simulink model "Rotor_Delevitation_PB_NonWhirl"  (R2024b)
settings: Solver=ode15s  StartTime=0.0  StopTime=.7  FixedStep=1e-4  MaxStep=1e-3  RelTol=1e-3  AbsTol=1e-3
undefined symbols (not defined in the file): points, X, x1, x2, x_i, x_o, Y, y_i, y_o, Z, z_i, z_o
libraries: sm_lib x361, nesl_utility x6
(part 4 of 6)

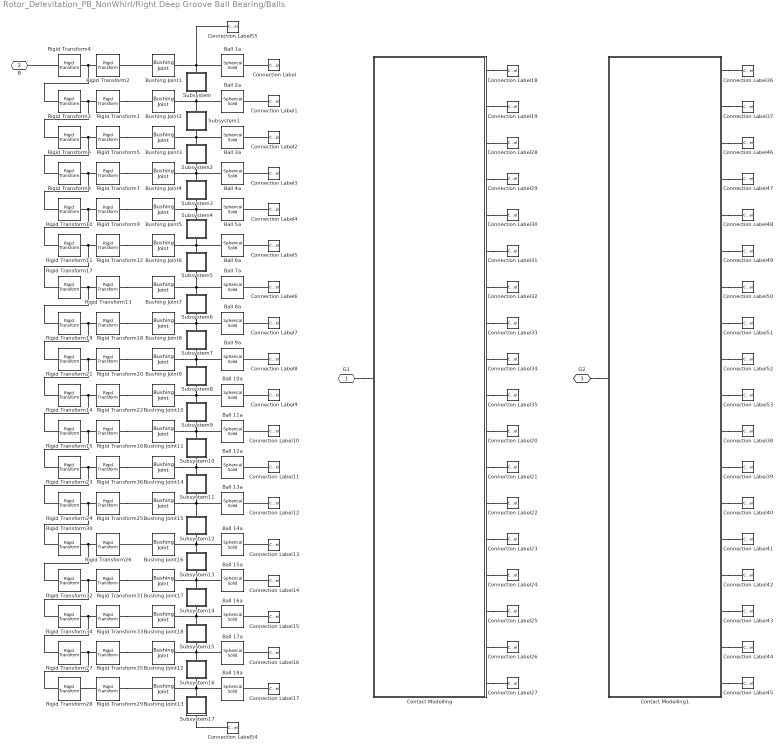
== system Rotor_Delevitation_PB_NonWhirl/Right Deep Groove Ball Bearing/Balls ==
  Ball 10a : sm_lib/Body Elements/Spherical Solid  SphereRadius=R-(C/2)  SphereRadiusUnits=mm  ExportEntireGeometry=on  InertiaType=CalculateFromGeometry  BasedOnType=Density  Density=1000  DensityUnits=kg/m^3  Mass=1  MassUnits=kg  CenterOfMass=[0 0 0]  CenterOfMassUnits=m  MomentsOfInertia=[1 1 1]  MomentsOfInertiaUnits=kg*m^2  ProductsOfInertia=[0 0 0]  ProductsOfInertiaUnits=kg*m^2  GraphicType=FromGeometry  MarkerShape=Sphere  MarkerSize=10  GraphicVisPropType=SimpleVisualProperties  GraphicDiffuseColor=[0.3922 0.8314 0.07451]  GraphicOpacity=1  GraphicSpecularColor=[0.5 0.5 0.5 1.0]  GraphicAmbientColor=[0.15 0.15 0.15 1.0]  GraphicEmissiveColor=[0.0 0.0 0.0 1.0]  GraphicShininess=75  DoExposeReferenceFrame=on  SerializedFrames=<Frames/>
  Ball 11a : sm_lib/Body Elements/Spherical Solid  SphereRadius=R-(C/2)  SphereRadiusUnits=mm  ExportEntireGeometry=on  InertiaType=CalculateFromGeometry  BasedOnType=Density  Density=1000  DensityUnits=kg/m^3  Mass=1  MassUnits=kg  CenterOfMass=[0 0 0]  CenterOfMassUnits=m  MomentsOfInertia=[1 1 1]  MomentsOfInertiaUnits=kg*m^2  ProductsOfInertia=[0 0 0]  ProductsOfInertiaUnits=kg*m^2  GraphicType=FromGeometry  MarkerShape=Sphere  MarkerSize=10  GraphicVisPropType=SimpleVisualProperties  GraphicDiffuseColor=[0.3922 0.8314 0.07451]  GraphicOpacity=1  GraphicSpecularColor=[0.5 0.5 0.5 1.0]  GraphicAmbientColor=[0.15 0.15 0.15 1.0]  GraphicEmissiveColor=[0.0 0.0 0.0 1.0]  GraphicShininess=75  DoExposeReferenceFrame=on  SerializedFrames=<Frames/>
  Ball 12a : sm_lib/Body Elements/Spherical Solid  SphereRadius=R-(C/2)  SphereRadiusUnits=mm  ExportEntireGeometry=on  InertiaType=CalculateFromGeometry  BasedOnType=Density  Density=1000  DensityUnits=kg/m^3  Mass=1  MassUnits=kg  CenterOfMass=[0 0 0]  CenterOfMassUnits=m  MomentsOfInertia=[1 1 1]  MomentsOfInertiaUnits=kg*m^2  ProductsOfInertia=[0 0 0]  ProductsOfInertiaUnits=kg*m^2  GraphicType=FromGeometry  MarkerShape=Sphere  MarkerSize=10  GraphicVisPropType=SimpleVisualProperties  GraphicDiffuseColor=[0.3922 0.8314 0.07451]  GraphicOpacity=1  GraphicSpecularColor=[0.5 0.5 0.5 1.0]  GraphicAmbientColor=[0.15 0.15 0.15 1.0]  GraphicEmissiveColor=[0.0 0.0 0.0 1.0]  GraphicShininess=75  DoExposeReferenceFrame=on  SerializedFrames=<Frames/>
  Ball 13a : sm_lib/Body Elements/Spherical Solid  SphereRadius=R-(C/2)  SphereRadiusUnits=mm  ExportEntireGeometry=on  InertiaType=CalculateFromGeometry  BasedOnType=Density  Density=1000  DensityUnits=kg/m^3  Mass=1  MassUnits=kg  CenterOfMass=[0 0 0]  CenterOfMassUnits=m  MomentsOfInertia=[1 1 1]  MomentsOfInertiaUnits=kg*m^2  ProductsOfInertia=[0 0 0]  ProductsOfInertiaUnits=kg*m^2  GraphicType=FromGeometry  MarkerShape=Sphere  MarkerSize=10  GraphicVisPropType=SimpleVisualProperties  GraphicDiffuseColor=[0.3922 0.8314 0.07451]  GraphicOpacity=1  GraphicSpecularColor=[0.5 0.5 0.5 1.0]  GraphicAmbientColor=[0.15 0.15 0.15 1.0]  GraphicEmissiveColor=[0.0 0.0 0.0 1.0]  GraphicShininess=75  DoExposeReferenceFrame=on  SerializedFrames=<Frames/>
  "Ball 14a " : sm_lib/Body Elements/Spherical Solid  SphereRadius=R-(C/2)  SphereRadiusUnits=mm  ExportEntireGeometry=on  InertiaType=CalculateFromGeometry  BasedOnType=Density  Density=1000  DensityUnits=kg/m^3  Mass=1  MassUnits=kg  CenterOfMass=[0 0 0]  CenterOfMassUnits=m  MomentsOfInertia=[1 1 1]  MomentsOfInertiaUnits=kg*m^2  ProductsOfInertia=[0 0 0]  ProductsOfInertiaUnits=kg*m^2  GraphicType=FromGeometry  MarkerShape=Sphere  MarkerSize=10  GraphicVisPropType=SimpleVisualProperties  GraphicDiffuseColor=[0.3922 0.8314 0.07451]  GraphicOpacity=1  GraphicSpecularColor=[0.5 0.5 0.5 1.0]  GraphicAmbientColor=[0.15 0.15 0.15 1.0]  GraphicEmissiveColor=[0.0 0.0 0.0 1.0]  GraphicShininess=75  DoExposeReferenceFrame=on  SerializedFrames=<Frames/>
  Ball 15a : sm_lib/Body Elements/Spherical Solid  SphereRadius=R-(C/2)  SphereRadiusUnits=mm  ExportEntireGeometry=on  InertiaType=CalculateFromGeometry  BasedOnType=Density  Density=1000  DensityUnits=kg/m^3  Mass=1  MassUnits=kg  CenterOfMass=[0 0 0]  CenterOfMassUnits=m  MomentsOfInertia=[1 1 1]  MomentsOfInertiaUnits=kg*m^2  ProductsOfInertia=[0 0 0]  ProductsOfInertiaUnits=kg*m^2  GraphicType=FromGeometry  MarkerShape=Sphere  MarkerSize=10  GraphicVisPropType=SimpleVisualProperties  GraphicDiffuseColor=[0.3922 0.8314 0.07451]  GraphicOpacity=1  GraphicSpecularColor=[0.5 0.5 0.5 1.0]  GraphicAmbientColor=[0.15 0.15 0.15 1.0]  GraphicEmissiveColor=[0.0 0.0 0.0 1.0]  GraphicShininess=75  DoExposeReferenceFrame=on  SerializedFrames=<Frames/>
  Ball 16a : sm_lib/Body Elements/Spherical Solid  SphereRadius=R-(C/2)  SphereRadiusUnits=mm  ExportEntireGeometry=on  InertiaType=CalculateFromGeometry  BasedOnType=Density  Density=1000  DensityUnits=kg/m^3  Mass=1  MassUnits=kg  CenterOfMass=[0 0 0]  CenterOfMassUnits=m  MomentsOfInertia=[1 1 1]  MomentsOfInertiaUnits=kg*m^2  ProductsOfInertia=[0 0 0]  ProductsOfInertiaUnits=kg*m^2  GraphicType=FromGeometry  MarkerShape=Sphere  MarkerSize=10  GraphicVisPropType=SimpleVisualProperties  GraphicDiffuseColor=[0.3922 0.8314 0.07451]  GraphicOpacity=1  GraphicSpecularColor=[0.5 0.5 0.5 1.0]  GraphicAmbientColor=[0.15 0.15 0.15 1.0]  GraphicEmissiveColor=[0.0 0.0 0.0 1.0]  GraphicShininess=75  DoExposeReferenceFrame=on  SerializedFrames=<Frames/>
  Ball 17a : sm_lib/Body Elements/Spherical Solid  SphereRadius=R-(C/2)  SphereRadiusUnits=mm  ExportEntireGeometry=on  InertiaType=CalculateFromGeometry  BasedOnType=Density  Density=1000  DensityUnits=kg/m^3  Mass=1  MassUnits=kg  CenterOfMass=[0 0 0]  CenterOfMassUnits=m  MomentsOfInertia=[1 1 1]  MomentsOfInertiaUnits=kg*m^2  ProductsOfInertia=[0 0 0]  ProductsOfInertiaUnits=kg*m^2  GraphicType=FromGeometry  MarkerShape=Sphere  MarkerSize=10  GraphicVisPropType=SimpleVisualProperties  GraphicDiffuseColor=[0.3922 0.8314 0.07451]  GraphicOpacity=1  GraphicSpecularColor=[0.5 0.5 0.5 1.0]  GraphicAmbientColor=[0.15 0.15 0.15 1.0]  GraphicEmissiveColor=[0.0 0.0 0.0 1.0]  GraphicShininess=75  DoExposeReferenceFrame=on  SerializedFrames=<Frames/>
  Ball 18a : sm_lib/Body Elements/Spherical Solid  SphereRadius=R-(C/2)  SphereRadiusUnits=mm  ExportEntireGeometry=on  InertiaType=CalculateFromGeometry  BasedOnType=Density  Density=1000  DensityUnits=kg/m^3  Mass=1  MassUnits=kg  CenterOfMass=[0 0 0]  CenterOfMassUnits=m  MomentsOfInertia=[1 1 1]  MomentsOfInertiaUnits=kg*m^2  ProductsOfInertia=[0 0 0]  ProductsOfInertiaUnits=kg*m^2  GraphicType=FromGeometry  MarkerShape=Sphere  MarkerSize=10  GraphicVisPropType=SimpleVisualProperties  GraphicDiffuseColor=[0.3922 0.8314 0.07451]  GraphicOpacity=1  GraphicSpecularColor=[0.5 0.5 0.5 1.0]  GraphicAmbientColor=[0.15 0.15 0.15 1.0]  GraphicEmissiveColor=[0.0 0.0 0.0 1.0]  GraphicShininess=75  DoExposeReferenceFrame=on  SerializedFrames=<Frames/>
  Ball 1a : sm_lib/Body Elements/Spherical Solid  SphereRadius=R-(C/2)  SphereRadiusUnits=mm  ExportEntireGeometry=on  InertiaType=CalculateFromGeometry  BasedOnType=Density  Density=1000  DensityUnits=kg/m^3  Mass=1  MassUnits=kg  CenterOfMass=[0 0 0]  CenterOfMassUnits=m  MomentsOfInertia=[1 1 1]  MomentsOfInertiaUnits=kg*m^2  ProductsOfInertia=[0 0 0]  ProductsOfInertiaUnits=kg*m^2  GraphicType=FromGeometry  MarkerShape=Sphere  MarkerSize=10  GraphicVisPropType=SimpleVisualProperties  GraphicDiffuseColor=[0.851 0.3255 0.09804]  GraphicOpacity=1  GraphicSpecularColor=[0.5 0.5 0.5 1.0]  GraphicAmbientColor=[0.15 0.15 0.15 1.0]  GraphicEmissiveColor=[0.0 0.0 0.0 1.0]  GraphicShininess=75  DoExposeReferenceFrame=on  SerializedFrames=<Frames/>
  Ball 2a : sm_lib/Body Elements/Spherical Solid  SphereRadius=R-(C/2)  SphereRadiusUnits=mm  ExportEntireGeometry=on  InertiaType=CalculateFromGeometry  BasedOnType=Density  Density=1000  DensityUnits=kg/m^3  Mass=1  MassUnits=kg  CenterOfMass=[0 0 0]  CenterOfMassUnits=m  MomentsOfInertia=[1 1 1]  MomentsOfInertiaUnits=kg*m^2  ProductsOfInertia=[0 0 0]  ProductsOfInertiaUnits=kg*m^2  GraphicType=FromGeometry  MarkerShape=Sphere  MarkerSize=10  GraphicVisPropType=SimpleVisualProperties  GraphicDiffuseColor=[0.3922 0.8314 0.07451]  GraphicOpacity=1  GraphicSpecularColor=[0.5 0.5 0.5 1.0]  GraphicAmbientColor=[0.15 0.15 0.15 1.0]  GraphicEmissiveColor=[0.0 0.0 0.0 1.0]  GraphicShininess=75  DoExposeReferenceFrame=on  SerializedFrames=<Frames/>
  Ball 3a : sm_lib/Body Elements/Spherical Solid  SphereRadius=R-(C/2)  SphereRadiusUnits=mm  ExportEntireGeometry=on  InertiaType=CalculateFromGeometry  BasedOnType=Density  Density=1000  DensityUnits=kg/m^3  Mass=1  MassUnits=kg  CenterOfMass=[0 0 0]  CenterOfMassUnits=m  MomentsOfInertia=[1 1 1]  MomentsOfInertiaUnits=kg*m^2  ProductsOfInertia=[0 0 0]  ProductsOfInertiaUnits=kg*m^2  GraphicType=FromGeometry  MarkerShape=Sphere  MarkerSize=10  GraphicVisPropType=SimpleVisualProperties  GraphicDiffuseColor=[0.3922 0.8314 0.07451]  GraphicOpacity=1  GraphicSpecularColor=[0.5 0.5 0.5 1.0]  GraphicAmbientColor=[0.15 0.15 0.15 1.0]  GraphicEmissiveColor=[0.0 0.0 0.0 1.0]  GraphicShininess=75  DoExposeReferenceFrame=on  SerializedFrames=<Frames/>
  Ball 4a : sm_lib/Body Elements/Spherical Solid  SphereRadius=R-(C/2)  SphereRadiusUnits=mm  ExportEntireGeometry=on  InertiaType=CalculateFromGeometry  BasedOnType=Density  Density=1000  DensityUnits=kg/m^3  Mass=1  MassUnits=kg  CenterOfMass=[0 0 0]  CenterOfMassUnits=m  MomentsOfInertia=[1 1 1]  MomentsOfInertiaUnits=kg*m^2  ProductsOfInertia=[0 0 0]  ProductsOfInertiaUnits=kg*m^2  GraphicType=FromGeometry  MarkerShape=Sphere  MarkerSize=10  GraphicVisPropType=SimpleVisualProperties  GraphicDiffuseColor=[0.3922 0.8314 0.07451]  GraphicOpacity=1  GraphicSpecularColor=[0.5 0.5 0.5 1.0]  GraphicAmbientColor=[0.15 0.15 0.15 1.0]  GraphicEmissiveColor=[0.0 0.0 0.0 1.0]  GraphicShininess=75  DoExposeReferenceFrame=on  SerializedFrames=<Frames/>
  Ball 5a : sm_lib/Body Elements/Spherical Solid  SphereRadius=R-(C/2)  SphereRadiusUnits=mm  ExportEntireGeometry=on  InertiaType=CalculateFromGeometry  BasedOnType=Density  Density=1000  DensityUnits=kg/m^3  Mass=1  MassUnits=kg  CenterOfMass=[0 0 0]  CenterOfMassUnits=m  MomentsOfInertia=[1 1 1]  MomentsOfInertiaUnits=kg*m^2  ProductsOfInertia=[0 0 0]  ProductsOfInertiaUnits=kg*m^2  GraphicType=FromGeometry  MarkerShape=Sphere  MarkerSize=10  GraphicVisPropType=SimpleVisualProperties  GraphicDiffuseColor=[0.3922 0.8314 0.07451]  GraphicOpacity=1  GraphicSpecularColor=[0.5 0.5 0.5 1.0]  GraphicAmbientColor=[0.15 0.15 0.15 1.0]  GraphicEmissiveColor=[0.0 0.0 0.0 1.0]  GraphicShininess=75  DoExposeReferenceFrame=on  SerializedFrames=<Frames/>
  "Ball 6a " : sm_lib/Body Elements/Spherical Solid  SphereRadius=R-(C/2)  SphereRadiusUnits=mm  ExportEntireGeometry=on  InertiaType=CalculateFromGeometry  BasedOnType=Density  Density=1000  DensityUnits=kg/m^3  Mass=1  MassUnits=kg  CenterOfMass=[0 0 0]  CenterOfMassUnits=m  MomentsOfInertia=[1 1 1]  MomentsOfInertiaUnits=kg*m^2  ProductsOfInertia=[0 0 0]  ProductsOfInertiaUnits=kg*m^2  GraphicType=FromGeometry  MarkerShape=Sphere  MarkerSize=10  GraphicVisPropType=SimpleVisualProperties  GraphicDiffuseColor=[0.3922 0.8314 0.07451]  GraphicOpacity=1  GraphicSpecularColor=[0.5 0.5 0.5 1.0]  GraphicAmbientColor=[0.15 0.15 0.15 1.0]  GraphicEmissiveColor=[0.0 0.0 0.0 1.0]  GraphicShininess=75  DoExposeReferenceFrame=on  SerializedFrames=<Frames/>
  Ball 7a : sm_lib/Body Elements/Spherical Solid  SphereRadius=R-(C/2)  SphereRadiusUnits=mm  ExportEntireGeometry=on  InertiaType=CalculateFromGeometry  BasedOnType=Density  Density=1000  DensityUnits=kg/m^3  Mass=1  MassUnits=kg  CenterOfMass=[0 0 0]  CenterOfMassUnits=m  MomentsOfInertia=[1 1 1]  MomentsOfInertiaUnits=kg*m^2  ProductsOfInertia=[0 0 0]  ProductsOfInertiaUnits=kg*m^2  GraphicType=FromGeometry  MarkerShape=Sphere  MarkerSize=10  GraphicVisPropType=SimpleVisualProperties  GraphicDiffuseColor=[0.3922 0.8314 0.07451]  GraphicOpacity=1  GraphicSpecularColor=[0.5 0.5 0.5 1.0]  GraphicAmbientColor=[0.15 0.15 0.15 1.0]  GraphicEmissiveColor=[0.0 0.0 0.0 1.0]  GraphicShininess=75  DoExposeReferenceFrame=on  SerializedFrames=<Frames/>
  Ball 8a : sm_lib/Body Elements/Spherical Solid  SphereRadius=R-(C/2)  SphereRadiusUnits=mm  ExportEntireGeometry=on  InertiaType=CalculateFromGeometry  BasedOnType=Density  Density=1000  DensityUnits=kg/m^3  Mass=1  MassUnits=kg  CenterOfMass=[0 0 0]  CenterOfMassUnits=m  MomentsOfInertia=[1 1 1]  MomentsOfInertiaUnits=kg*m^2  ProductsOfInertia=[0 0 0]  ProductsOfInertiaUnits=kg*m^2  GraphicType=FromGeometry  MarkerShape=Sphere  MarkerSize=10  GraphicVisPropType=SimpleVisualProperties  GraphicDiffuseColor=[0.3922 0.8314 0.07451]  GraphicOpacity=1  GraphicSpecularColor=[0.5 0.5 0.5 1.0]  GraphicAmbientColor=[0.15 0.15 0.15 1.0]  GraphicEmissiveColor=[0.0 0.0 0.0 1.0]  GraphicShininess=75  DoExposeReferenceFrame=on  SerializedFrames=<Frames/>
  Ball 9a : sm_lib/Body Elements/Spherical Solid  SphereRadius=R-(C/2)  SphereRadiusUnits=mm  ExportEntireGeometry=on  InertiaType=CalculateFromGeometry  BasedOnType=Density  Density=1000  DensityUnits=kg/m^3  Mass=1  MassUnits=kg  CenterOfMass=[0 0 0]  CenterOfMassUnits=m  MomentsOfInertia=[1 1 1]  MomentsOfInertiaUnits=kg*m^2  ProductsOfInertia=[0 0 0]  ProductsOfInertiaUnits=kg*m^2  GraphicType=FromGeometry  MarkerShape=Sphere  MarkerSize=10  GraphicVisPropType=SimpleVisualProperties  GraphicDiffuseColor=[0.3922 0.8314 0.07451]  GraphicOpacity=1  GraphicSpecularColor=[0.5 0.5 0.5 1.0]  GraphicAmbientColor=[0.15 0.15 0.15 1.0]  GraphicEmissiveColor=[0.0 0.0 0.0 1.0]  GraphicShininess=75  DoExposeReferenceFrame=on  SerializedFrames=<Frames/>
  Bushing Joint{1..18} (18 alike) : sm_lib/Joints/Bushing Joint  JointMode=Normal  CompositeWrenchDir=FollowerOnBase  CompositeWrenchFrame=BaseFrame  SenseConstraintForce=off  SenseConstraintTorque=off  SenseTotalForce=off  SenseTotalTorque=off  PxPositionTargetSpecify=off  PxPositionTargetPriority=High  PxPositionTargetValue=0  PxPositionTargetValueUnits=m  PxVelocityTargetSpecify=off  PxVelocityTargetPriority=High  PxVelocityTargetValue=0  PxVelocityTargetValueUnits=m/s  PxEquilibriumPosition=0  PxEquilibriumPositionUnits=m  PxSpringStiffness=0  PxSpringStiffnessUnits=N/m  PxDampingCoefficient=0  PxDampingCoefficientUnits=N/(m/s)  PxLowerLimitSpecify=off  PxLowerLimitBound=-1  PxLowerLimitBoundUnits=m  PxLowerLimitStiffness=1e6  PxLowerLimitStiffnessUnits=N/m  PxLowerLimitDamping=1e3  PxLowerLimitDampingUnits=N/(m/s)  PxLowerLimitTransitionRegionWidth=1e-4  PxLowerLimitTransitionRegionWidthUnits=m  PxUpperLimitSpecify=off  PxUpperLimitBound=1  PxUpperLimitBoundUnits=m  PxUpperLimitStiffness=1e6  PxUpperLimitStiffnessUnits=N/m  PxUpperLimitDamping=1e3  PxUpperLimitDampingUnits=N/(m/s)  PxUpperLimitTransitionRegionWidth=1e-4  PxUpperLimitTransitionRegionWidthUnits=m  PxTorqueActuationMode=NoTorque  PxMotionActuationMode=ComputedMotion  PxSensePosition=off  PxSenseVelocity=off  PxSenseAcceleration=off  PxSenseTorqueForce=off  PxSenseLowerLimitTorqueForce=off  PxSenseUpperLimitTorqueForce=off  PyPositionTargetSpecify=off  PyPositionTargetPriority=High  PyPositionTargetValue=0  PyPositionTargetValueUnits=m  PyVelocityTargetSpecify=off  PyVelocityTargetPriority=High  PyVelocityTargetValue=0  PyVelocityTargetValueUnits=m/s  PyEquilibriumPosition=0  PyEquilibriumPositionUnits=m  PySpringStiffness=0  PySpringStiffnessUnits=N/m  PyDampingCoefficient=0  PyDampingCoefficientUnits=N/(m/s)  PyLowerLimitSpecify=off  PyLowerLimitBound=-1  PyLowerLimitBoundUnits=m  PyLowerLimitStiffness=1e6  PyLowerLimitStiffnessUnits=N/m  PyLowerLimitDamping=1e3  PyLowerLimitDampingUnits=N/(m/s)  PyLowerLimitTransitionRegionWidth=1e-4  PyLowerLimitTransitionRegionWidthUnits=m  PyUpperLimitSpecify=off  PyUpperLimitBound=1  PyUpperLimitBoundUnits=m  PyUpperLimitStiffness=1e6  PyUpperLimitStiffnessUnits=N/m  PyUpperLimitDamping=1e3  PyUpperLimitDampingUnits=N/(m/s)  PyUpperLimitTransitionRegionWidth=1e-4  PyUpperLimitTransitionRegionWidthUnits=m  PyTorqueActuationMode=NoTorque  PyMotionActuationMode=ComputedMotion  PySensePosition=off  PySenseVelocity=off  PySenseAcceleration=off  PySenseTorqueForce=off  PySenseLowerLimitTorqueForce=off  PySenseUpperLimitTorqueForce=off  PzPositionTargetSpecify=off  PzPositionTargetPriority=High  PzPositionTargetValue=0  PzPositionTargetValueUnits=m  PzVelocityTargetSpecify=off  PzVelocityTargetPriority=High  PzVelocityTargetValue=0  PzVelocityTargetValueUnits=m/s  PzEquilibriumPosition=0  PzEquilibriumPositionUnits=m  PzSpringStiffness=0  PzSpringStiffnessUnits=N/m  PzDampingCoefficient=0  PzDampingCoefficientUnits=N/(m/s)  PzLowerLimitSpecify=off  PzLowerLimitBound=-1  PzLowerLimitBoundUnits=m  PzLowerLimitStiffness=1e6  PzLowerLimitStiffnessUnits=N/m  PzLowerLimitDamping=1e3  PzLowerLimitDampingUnits=N/(m/s)  PzLowerLimitTransitionRegionWidth=1e-4  PzLowerLimitTransitionRegionWidthUnits=m  PzUpperLimitSpecify=off  PzUpperLimitBound=1  PzUpperLimitBoundUnits=m  PzUpperLimitStiffness=1e6  PzUpperLimitStiffnessUnits=N/m  PzUpperLimitDamping=1e3  PzUpperLimitDampingUnits=N/(m/s)  PzUpperLimitTransitionRegionWidth=1e-4  PzUpperLimitTransitionRegionWidthUnits=m  PzTorqueActuationMode=NoTorque  PzMotionActuationMode=ComputedMotion  PzSensePosition=off  PzSenseVelocity=off  PzSenseAcceleration=off  PzSenseTorqueForce=off  PzSenseLowerLimitTorqueForce=off  PzSenseUpperLimitTorqueForce=off  RxPositionTargetSpecify=off  RxPositionTargetPriority=High  RxPositionTargetValue=0  RxPositionTargetValueUnits=deg  RxVelocityTargetSpecify=off  RxVelocityTargetPriority=High  RxVelocityTargetValue=0  RxVelocityTargetValueUnits=deg/s  RxEquilibriumPosition=0  RxEquilibriumPositionUnits=deg  RxSpringStiffness=0  RxSpringStiffnessUnits=N*m/deg  RxDampingCoefficient=0  RxDampingCoefficientUnits=N*m/(deg/s)  RxLowerLimitSpecify=off  RxLowerLimitBound=-90  RxLowerLimitBoundUnits=deg  RxLowerLimitStiffness=1e4  RxLowerLimitStiffnessUnits=N*m/deg  RxLowerLimitDamping=10  RxLowerLimitDampingUnits=N*m/(deg/s)  RxLowerLimitTransitionRegionWidth=0.1  RxLowerLimitTransitionRegionWidthUnits=deg  RxUpperLimitSpecify=off  RxUpperLimitBound=90  RxUpperLimitBoundUnits=deg  RxUpperLimitStiffness=1e4  RxUpperLimitStiffnessUnits=N*m/deg  RxUpperLimitDamping=10  RxUpperLimitDampingUnits=N*m/(deg/s)  RxUpperLimitTransitionRegionWidth=0.1  RxUpperLimitTransitionRegionWidthUnits=deg  RxTorqueActuationMode=NoTorque  RxMotionActuationMode=ComputedMotion  RxSensePosition=off  RxSenseVelocity=off  RxSenseAcceleration=off  RxSenseTorqueForce=off  RxSenseLowerLimitTorqueForce=off  RxSenseUpperLimitTorqueForce=off  RyPositionTargetSpecify=off  RyPositionTargetPriority=High  RyPositionTargetValue=0  RyPositionTargetValueUnits=deg  RyVelocityTargetSpecify=off  RyVelocityTargetPriority=High  RyVelocityTargetValue=0  RyVelocityTargetValueUnits=deg/s  RyEquilibriumPosition=0  RyEquilibriumPositionUnits=deg  RySpringStiffness=0  RySpringStiffnessUnits=N*m/deg  RyDampingCoefficient=0  RyDampingCoefficientUnits=N*m/(deg/s)  RyLowerLimitSpecify=off  RyLowerLimitBound=-90  RyLowerLimitBoundUnits=deg  RyLowerLimitStiffness=1e4  RyLowerLimitStiffnessUnits=N*m/deg  RyLowerLimitDamping=10  RyLowerLimitDampingUnits=N*m/(deg/s)  RyLowerLimitTransitionRegionWidth=0.1  RyLowerLimitTransitionRegionWidthUnits=deg  RyUpperLimitSpecify=off  RyUpperLimitBound=90  RyUpperLimitBoundUnits=deg  RyUpperLimitStiffness=1e4  RyUpperLimitStiffnessUnits=N*m/deg  RyUpperLimitDamping=10  RyUpperLimitDampingUnits=N*m/(deg/s)  RyUpperLimitTransitionRegionWidth=0.1  RyUpperLimitTransitionRegionWidthUnits=deg  RyTorqueActuationMode=NoTorque  RyMotionActuationMode=ComputedMotion  RySensePosition=off  RySenseVelocity=off  RySenseAcceleration=off  RySenseTorqueForce=off  RySenseLowerLimitTorqueForce=off  RySenseUpperLimitTorqueForce=off  RzPositionTargetSpecify=off  RzPositionTargetPriority=High  RzPositionTargetValue=0  RzPositionTargetValueUnits=deg  RzVelocityTargetSpecify=off  RzVelocityTargetPriority=High  RzVelocityTargetValue=0  RzVelocityTargetValueUnits=deg/s  RzEquilibriumPosition=0  RzEquilibriumPositionUnits=deg  RzSpringStiffness=0  RzSpringStiffnessUnits=N*m/deg  RzDampingCoefficient=0  RzDampingCoefficientUnits=N*m/(deg/s)  RzLowerLimitSpecify=off  RzLowerLimitBound=-90  RzLowerLimitBoundUnits=deg  RzLowerLimitStiffness=1e4  RzLowerLimitStiffnessUnits=N*m/deg  RzLowerLimitDamping=10  RzLowerLimitDampingUnits=N*m/(deg/s)  RzLowerLimitTransitionRegionWidth=0.1  RzLowerLimitTransitionRegionWidthUnits=deg  RzUpperLimitSpecify=off  RzUpperLimitBound=90  RzUpperLimitBoundUnits=deg  RzUpperLimitStiffness=1e4  RzUpperLimitStiffnessUnits=N*m/deg  RzUpperLimitDamping=10  RzUpperLimitDampingUnits=N*m/(deg/s)  RzUpperLimitTransitionRegionWidth=0.1  RzUpperLimitTransitionRegionWidthUnits=deg  RzTorqueActuationMode=NoTorque  RzMotionActuationMode=ComputedMotion  RzSensePosition=off  RzSenseVelocity=off  RzSenseAcceleration=off  RzSenseTorqueForce=off  RzSenseLowerLimitTorqueForce=off  RzSenseUpperLimitTorqueForce=off
  Connection Label : ConnectionLabel
  Connection Label1 : ConnectionLabel  Label=Label2
  Connection Label10 : ConnectionLabel  Label=Label11
  Connection Label11 : ConnectionLabel  Label=Label12
  Connection Label12 : ConnectionLabel  Label=Label13
  Connection Label13 : ConnectionLabel  Label=Label14
  Connection Label14 : ConnectionLabel  Label=Label15
  Connection Label15 : ConnectionLabel  Label=Label16
  Connection Label16 : ConnectionLabel  Label=Label17
  Connection Label17 : ConnectionLabel  Label=Label18
  Connection Label18 : ConnectionLabel
  Connection Label19 : ConnectionLabel  Label=Label2
  Connection Label2 : ConnectionLabel  Label=Label3
  Connection Label20 : ConnectionLabel  Label=Label11
  Connection Label21 : ConnectionLabel  Label=Label12
  Connection Label22 : ConnectionLabel  Label=Label13
  Connection Label23 : ConnectionLabel  Label=Label14
  Connection Label24 : ConnectionLabel  Label=Label15
  Connection Label25 : ConnectionLabel  Label=Label16
  Connection Label26 : ConnectionLabel  Label=Label17
  Connection Label27 : ConnectionLabel  Label=Label18
  Connection Label28 : ConnectionLabel  Label=Label3
  Connection Label29 : ConnectionLabel  Label=Label4
  Connection Label3 : ConnectionLabel  Label=Label4
  Connection Label30 : ConnectionLabel  Label=Label5
  Connection Label31 : ConnectionLabel  Label=Label6
  Connection Label32 : ConnectionLabel  Label=Label7
  Connection Label33 : ConnectionLabel  Label=Label8
  Connection Label34 : ConnectionLabel  Label=Label9
  Connection Label35 : ConnectionLabel  Label=Label10
  Connection Label36 : ConnectionLabel
  Connection Label37 : ConnectionLabel  Label=Label2
  Connection Label38 : ConnectionLabel  Label=Label11
  Connection Label39 : ConnectionLabel  Label=Label12
  Connection Label4 : ConnectionLabel  Label=Label5
  Connection Label40 : ConnectionLabel  Label=Label13
  Connection Label41 : ConnectionLabel  Label=Label14
  Connection Label42 : ConnectionLabel  Label=Label15
  Connection Label43 : ConnectionLabel  Label=Label16
  Connection Label44 : ConnectionLabel  Label=Label17
  Connection Label45 : ConnectionLabel  Label=Label18
  Connection Label46 : ConnectionLabel  Label=Label3
  Connection Label47 : ConnectionLabel  Label=Label4
  Connection Label48 : ConnectionLabel  Label=Label5
  Connection Label49 : ConnectionLabel  Label=Label6
  Connection Label5 : ConnectionLabel  Label=Label6
  Connection Label50 : ConnectionLabel  Label=Label7
  Connection Label51 : ConnectionLabel  Label=Label8
  Connection Label52 : ConnectionLabel  Label=Label9
  Connection Label53 : ConnectionLabel  Label=Label10
  Connection Label54 : ConnectionLabel  Label=Ball2Ball
  Connection Label55 : ConnectionLabel  Label=Ball2Ball
  Connection Label6 : ConnectionLabel  Label=Label7
  Connection Label7 : ConnectionLabel  Label=Label8
  Connection Label8 : ConnectionLabel  Label=Label9
  Connection Label9 : ConnectionLabel  Label=Label10
  Contact Modelling : Subsystem
  Contact Modelling1 : Subsystem
  Rigid Transform{1,5,7,9,12..13,16,18,20,22,25..26,29,31,33,35..36} (17 alike) : sm_lib/Frames and Transforms/Rigid Transform  RotationMethod=None  FollAlignAxisA=+X  BaseAlignAxisA=+Y  FollAlignAxisB=+Y  BaseAlignAxisB=+Z  RotationStandardAxis=+X  RotationAngle=20  RotationAngleUnits=deg  RotationArbitraryAxis=[0 0 1]  RotationSequenceAxes=FollowerAxes  RotationSequence=XYX  RotationSequenceAngles=[0 0 0]  RotationSequenceAnglesUnits=deg  RotationMatrix=[1 0 0;0 1 0;0 0 1]  Quaternion=[1 0 0 0]  TranslationMethod=Cartesian  TranslationCartesianOffset=-[0 (ROO+RII)/2 0]  TranslationCartesianOffsetUnits=mm  TranslationStandardAxis=+Z  TranslationStandardOffset=0  TranslationStandardOffsetUnits=m  TranslationROffset=0  TranslationROffsetUnits=m  TranslationThetaOffset=0  TranslationThetaOffsetUnits=deg  TranslationZOffset=0  TranslationZOffsetUnits=m
  Rigid Transform{3,6,8,10..11,14..15,17,19,21,23..24,27..28,30,32,34} (17 alike) : sm_lib/Frames and Transforms/Rigid Transform  RotationMethod=StandardAxis  FollAlignAxisA=+X  BaseAlignAxisA=+Y  FollAlignAxisB=+Y  BaseAlignAxisB=+Z  RotationStandardAxis=+Z  RotationAngle=20  RotationAngleUnits=deg  RotationArbitraryAxis=[0 0 1]  RotationSequenceAxes=FollowerAxes  RotationSequence=XYX  RotationSequenceAngles=[0 0 0]  RotationSequenceAnglesUnits=deg  RotationMatrix=[1 0 0;0 1 0;0 0 1]  Quaternion=[1 0 0 0]  TranslationMethod=None  TranslationCartesianOffset=-[0 (ROO+RII)/2 0]  TranslationCartesianOffsetUnits=mm  TranslationStandardAxis=+Z  TranslationStandardOffset=0  TranslationStandardOffsetUnits=m  TranslationROffset=0  TranslationROffsetUnits=m  TranslationThetaOffset=0  TranslationThetaOffsetUnits=deg  TranslationZOffset=0  TranslationZOffsetUnits=m
  Rigid Transform2 : sm_lib/Frames and Transforms/Rigid Transform  RotationMethod=None  FollAlignAxisA=+X  BaseAlignAxisA=+Y  FollAlignAxisB=+Y  BaseAlignAxisB=+Z  RotationStandardAxis=+Z  RotationAngle=0  RotationAngleUnits=deg  RotationArbitraryAxis=[0 0 1]  RotationSequenceAxes=FollowerAxes  RotationSequence=XYX  RotationSequenceAngles=[0 0 0]  RotationSequenceAnglesUnits=deg  RotationMatrix=[1 0 0;0 1 0;0 0 1]  Quaternion=[1 0 0 0]  TranslationMethod=Cartesian  TranslationCartesianOffset=-[0 (ROO+RII)/2 0]  TranslationCartesianOffsetUnits=mm  TranslationStandardAxis=+Z  TranslationStandardOffset=0  TranslationStandardOffsetUnits=m  TranslationROffset=0  TranslationROffsetUnits=m  TranslationThetaOffset=0  TranslationThetaOffsetUnits=deg  TranslationZOffset=0  TranslationZOffsetUnits=m
  Rigid Transform4 : sm_lib/Frames and Transforms/Rigid Transform  RotationMethod=StandardAxis  FollAlignAxisA=+X  BaseAlignAxisA=+Y  FollAlignAxisB=+Y  BaseAlignAxisB=+Z  RotationStandardAxis=+Z  RotationAngle=0  RotationAngleUnits=deg  RotationArbitraryAxis=[0 0 1]  RotationSequenceAxes=FollowerAxes  RotationSequence=XYX  RotationSequenceAngles=[0 0 0]  RotationSequenceAnglesUnits=deg  RotationMatrix=[1 0 0;0 1 0;0 0 1]  Quaternion=[1 0 0 0]  TranslationMethod=None  TranslationCartesianOffset=-[0 (ROO+RII)/2 0]  TranslationCartesianOffsetUnits=mm  TranslationStandardAxis=+Z  TranslationStandardOffset=0  TranslationStandardOffsetUnits=m  TranslationROffset=0  TranslationROffsetUnits=m  TranslationThetaOffset=0  TranslationThetaOffsetUnits=deg  TranslationZOffset=0  TranslationZOffsetUnits=m
  Subsystem : Subsystem
  Subsystem1 : Subsystem
  Subsystem10 : Subsystem
  Subsystem11 : Subsystem
  Subsystem12 : Subsystem
  Subsystem13 : Subsystem
  Subsystem14 : Subsystem
  Subsystem15 : Subsystem
  Subsystem16 : Subsystem
  Subsystem17 : Subsystem
  Subsystem2 : Subsystem
  Subsystem3 : Subsystem
  Subsystem4 : Subsystem
  Subsystem5 : Subsystem
  Subsystem6 : Subsystem
  Subsystem7 : Subsystem
  Subsystem8 : Subsystem
  Subsystem9 : Subsystem
  G1 : PMIOPort  Side=Right
  B : PMIOPort  Port=2  Side=Left
  G2 : PMIOPort  Port=3  Side=Right
  connections:
  Subsystem17/RConn1 -- Connection Label54/LConn1
  Connection Label3/LConn1 -- Ball 4a/LConn1
  Contact Modelling1/RConn14 -- Connection Label41/LConn1
  G2/RConn1 -- Contact Modelling1/LConn1
  Contact Modelling1/RConn12 -- Connection Label39/LConn1
  Contact Modelling1/RConn13 -- Connection Label40/LConn1
  Contact Modelling1/RConn7 -- Connection Label50/LConn1
  Contact Modelling1/RConn18 -- Connection Label45/LConn1
  Contact Modelling1/RConn17 -- Connection Label44/LConn1
  Contact Modelling1/RConn11 -- Connection Label38/LConn1
  Contact Modelling1/RConn9 -- Connection Label52/LConn1
  Contact Modelling1/RConn8 -- Connection Label51/LConn1
  Contact Modelling1/RConn3 -- Connection Label46/LConn1
  Contact Modelling1/RConn5 -- Connection Label48/LConn1
  Contact Modelling1/RConn2 -- Connection Label37/LConn1
  Contact Modelling1/RConn10 -- Connection Label53/LConn1
  Contact Modelling1/RConn15 -- Connection Label42/LConn1
  Contact Modelling1/RConn1 -- Connection Label36/LConn1
  Contact Modelling1/RConn4 -- Connection Label47/LConn1
  Contact Modelling1/RConn16 -- Connection Label43/LConn1
  Contact Modelling1/RConn6 -- Connection Label49/LConn1
  Contact Modelling/RConn11 -- Connection Label20/LConn1
  Contact Modelling/RConn6 -- Connection Label31/LConn1
  Contact Modelling/RConn16 -- Connection Label25/LConn1
  Contact Modelling/RConn4 -- Connection Label29/LConn1
  Contact Modelling/RConn1 -- Connection Label18/LConn1
  Contact Modelling/RConn15 -- Connection Label24/LConn1
  Contact Modelling/RConn10 -- Connection Label35/LConn1
  Contact Modelling/RConn2 -- Connection Label19/LConn1
  Contact Modelling/RConn5 -- Connection Label30/LConn1
  Contact Modelling/RConn3 -- Connection Label28/LConn1
  Contact Modelling/RConn8 -- Connection Label33/LConn1
  Contact Modelling/RConn9 -- Connection Label34/LConn1
  Contact Modelling/RConn17 -- Connection Label26/LConn1
  Contact Modelling/RConn18 -- Connection Label27/LConn1
  Contact Modelling/RConn12 -- Connection Label21/LConn1
  Contact Modelling/RConn13 -- Connection Label22/LConn1
  Contact Modelling/RConn7 -- Connection Label32/LConn1
  Contact Modelling/RConn14 -- Connection Label23/LConn1
  G1/RConn1 -- Contact Modelling/LConn1
  Rigid Transform32/LConn1 -- Rigid Transform30/RConn1 -- Rigid Transform26/LConn1
  Bushing Joint16/LConn1 -- Rigid Transform26/RConn1
  Subsystem13/LConn1 -- "Ball 14a "/RConn1 -- Bushing Joint16/RConn1 -- Subsystem12/RConn1
  Connection Label13/LConn1 -- "Ball 14a "/LConn1
  Connection Label6/LConn1 -- Ball 7a/LConn1
  Subsystem6/LConn1 -- Ball 7a/RConn1 -- Bushing Joint7/RConn1 -- Subsystem5/RConn1
  Rigid Transform19/LConn1 -- Rigid Transform17/RConn1 -- Rigid Transform13/LConn1
  Rigid Transform13/RConn1 -- Bushing Joint7/LConn1
  Connection Label12/LConn1 -- Ball 13a/LConn1
  Rigid Transform24/LConn1 -- Rigid Transform36/LConn1 -- Rigid Transform23/RConn1
  Subsystem11/LConn1 -- Ball 12a/RConn1 -- Bushing Joint14/RConn1 -- Subsystem10/RConn1
  Connection Label11/LConn1 -- Ball 12a/LConn1
  Rigid Transform25/RConn1 -- Bushing Joint15/LConn1
  Rigid Transform36/RConn1 -- Bushing Joint14/LConn1
  Subsystem12/LConn1 -- Ball 13a/RConn1 -- Bushing Joint15/RConn1 -- Subsystem11/RConn1
  Rigid Transform30/LConn1 -- Rigid Transform25/LConn1 -- Rigid Transform24/RConn1
  Rigid Transform29/LConn1 -- Rigid Transform28/RConn1
  Subsystem17/LConn1 -- Ball 18a/RConn1 -- Bushing Joint13/RConn1 -- Subsystem16/RConn1
  Rigid Transform34/LConn1 -- Rigid Transform31/LConn1 -- Rigid Transform32/RConn1
  Connection Label17/LConn1 -- Ball 18a/LConn1
  Rigid Transform29/RConn1 -- Bushing Joint13/LConn1
  Rigid Transform28/LConn1 -- Rigid Transform35/LConn1 -- Rigid Transform27/RConn1
  Rigid Transform35/RConn1 -- Bushing Joint12/LConn1
  Connection Label16/LConn1 -- Ball 17a/LConn1
  Subsystem16/LConn1 -- Ball 17a/RConn1 -- Bushing Joint12/RConn1 -- Subsystem15/RConn1
  Rigid Transform27/LConn1 -- Rigid Transform33/LConn1 -- Rigid Transform34/RConn1
  Subsystem15/LConn1 -- Ball 16a/RConn1 -- Bushing Joint18/RConn1 -- Subsystem14/RConn1
  Connection Label14/LConn1 -- Ball 15a/LConn1
  Subsystem14/LConn1 -- Ball 15a/RConn1 -- Bushing Joint17/RConn1 -- Subsystem13/RConn1
  Rigid Transform31/RConn1 -- Bushing Joint17/LConn1
  Connection Label15/LConn1 -- Ball 16a/LConn1
  Rigid Transform33/RConn1 -- Bushing Joint18/LConn1
  Rigid Transform21/LConn1 -- Rigid Transform18/LConn1 -- Rigid Transform19/RConn1
  Rigid Transform20/RConn1 -- Bushing Joint9/LConn1
  Connection Label8/LConn1 -- Ball 9a/LConn1
  Rigid Transform18/RConn1 -- Bushing Joint8/LConn1
  Subsystem7/LConn1 -- Ball 8a/RConn1 -- Bushing Joint8/RConn1 -- Subsystem6/RConn1
  Connection Label7/LConn1 -- Ball 8a/LConn1
  Subsystem8/LConn1 -- Ball 9a/RConn1 -- Bushing Joint9/RConn1 -- Subsystem7/RConn1
  Rigid Transform14/LConn1 -- Rigid Transform20/LConn1 -- Rigid Transform21/RConn1
  Rigid Transform15/LConn1 -- Rigid Transform22/LConn1 -- Rigid Transform14/RConn1
  Subsystem9/LConn1 -- Ball 10a/RConn1 -- Bushing Joint10/RConn1 -- Subsystem8/RConn1
  Connection Label9/LConn1 -- Ball 10a/LConn1
  Rigid Transform22/RConn1 -- Bushing Joint10/LConn1
  Rigid Transform16/RConn1 -- Bushing Joint11/LConn1
  Connection Label10/LConn1 -- Ball 11a/LConn1
  Subsystem10/LConn1 -- Ball 11a/RConn1 -- Bushing Joint11/RConn1 -- Subsystem9/RConn1
  Rigid Transform23/LConn1 -- Rigid Transform16/LConn1 -- Rigid Transform15/RConn1
  Rigid Transform17/LConn1 -- Rigid Transform12/LConn1 -- Rigid Transform11/RConn1
  Subsystem5/LConn1 -- "Ball 6a "/RConn1 -- Bushing Joint6/RConn1 -- Subsystem4/RConn1
  Connection Label5/LConn1 -- "Ball 6a "/LConn1
  Rigid Transform12/RConn1 -- Bushing Joint6/LConn1
  Rigid Transform9/RConn1 -- Bushing Joint5/LConn1
  Connection Label4/LConn1 -- Ball 5a/LConn1
  Subsystem4/LConn1 -- Ball 5a/RConn1 -- Bushing Joint5/RConn1 -- Subsystem3/RConn1
  Rigid Transform11/LConn1 -- Rigid Transform9/LConn1 -- Rigid Transform10/RConn1
  Rigid Transform7/RConn1 -- Bushing Joint4/LConn1
  Rigid Transform10/LConn1 -- Rigid Transform7/LConn1 -- Rigid Transform8/RConn1
  Subsystem3/LConn1 -- Ball 4a/RConn1 -- Bushing Joint4/RConn1 -- Subsystem2/RConn1
  Connection Label2/LConn1 -- Ball 3a/LConn1
  Rigid Transform5/RConn1 -- Bushing Joint3/LConn1
  Subsystem2/LConn1 -- Ball 3a/RConn1 -- Bushing Joint3/RConn1 -- Subsystem1/RConn1
  Rigid Transform8/LConn1 -- Rigid Transform5/LConn1 -- Rigid Transform6/RConn1
  Rigid Transform3/LConn1 -- Rigid Transform2/LConn1 -- Rigid Transform4/RConn1
  Subsystem1/LConn1 -- Ball 2a/RConn1 -- Subsystem/RConn1 -- Bushing Joint2/RConn1
  Rigid Transform6/LConn1 -- Rigid Transform1/LConn1 -- Rigid Transform3/RConn1
  Rigid Transform1/RConn1 -- Bushing Joint2/LConn1
  Connection Label1/LConn1 -- Ball 2a/LConn1
  Connection Label/LConn1 -- Ball 1a/LConn1
  Connection Label55/LConn1 -- Ball 1a/RConn1 -- Subsystem/LConn1 -- Bushing Joint1/RConn1
  Bushing Joint1/LConn1 -- Rigid Transform2/RConn1
  Rigid Transform4/LConn1 -- B/RConn1

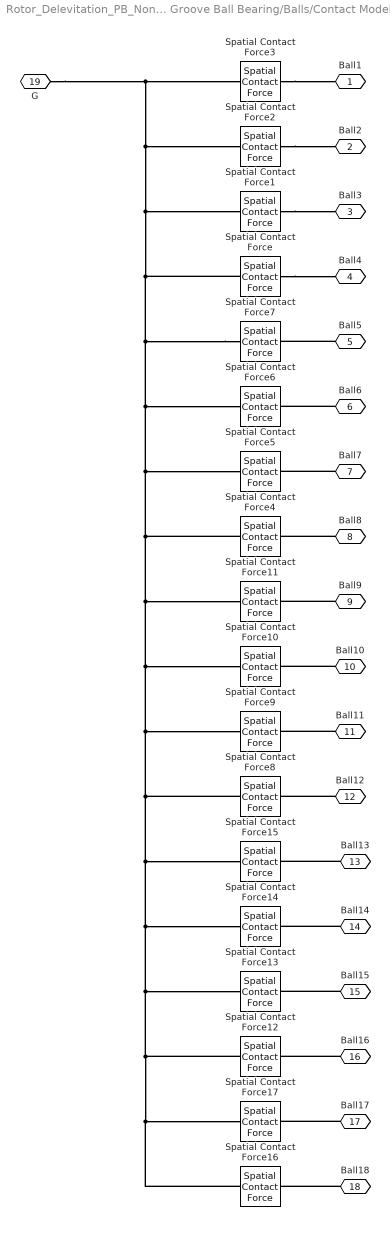
== system Rotor_Delevitation_PB_NonWhirl/Left Deep Groove Ball Bearing/Balls/Contact Modelling ==
  Spatial Contact Force{,1..17} (18 alike) : sm_lib/Forces and Torques/Spatial Contact Force  NormalForceType=SmoothSpringDamper  NormalStiffness=1e6  NormalStiffnessUnits=N/m  NormalDamping=1e3  NormalDampingUnits=N/(m/s)  NormalTransitionRegionWidth=1e-4  NormalTransitionRegionWidthUnits=m  FrictionType=SmoothStickSlip  CoefficientOfStaticFriction=0.5  CoefficientOfDynamicFriction=0.3  FrictionalCriticalVelocity=1e-3  FrictionalCriticalVelocityUnits=m/s  SenseContactSignal=off  SensePenetrationDepth=off  SenseSeparationDistance=off  SenseNormalForceMagnitude=off  SenseFrictionalForceMagnitude=off  SenseNormalVelocity=off  SenseTangentialVelocity=off  SenseContactBaseRotation=off  SenseContactBaseTranslation=off  SenseContactFollowerRotation=off  SenseContactFollowerTranslation=off  ZeroCrossDetectContactStartAndEnd=off
  Ball1 : PMIOPort  Side=Right
  Ball2 : PMIOPort  Port=2  Side=Right
  Ball3 : PMIOPort  Port=3  Side=Right
  Ball4 : PMIOPort  Port=4  Side=Right
  Ball5 : PMIOPort  Port=5  Side=Right
  Ball6 : PMIOPort  Port=6  Side=Right
  Ball7 : PMIOPort  Port=7  Side=Right
  Ball8 : PMIOPort  Port=8  Side=Right
  Ball9 : PMIOPort  Port=9  Side=Right
  Ball10 : PMIOPort  Port=10  Side=Right
  Ball11 : PMIOPort  Port=11  Side=Right
  Ball12 : PMIOPort  Port=12  Side=Right
  Ball13 : PMIOPort  Port=13  Side=Right
  Ball14 : PMIOPort  Port=14  Side=Right
  Ball15 : PMIOPort  Port=15  Side=Right
  Ball16 : PMIOPort  Port=16  Side=Right
  Ball17 : PMIOPort  Port=17  Side=Right
  Ball18 : PMIOPort  Port=18  Side=Right
  G : PMIOPort  Port=19  Side=Left
  connections:
  Spatial Contact Force2/LConn1 -- Ball2/RConn1
  Spatial Contact Force/LConn1 -- Ball4/RConn1
  Spatial Contact Force1/LConn1 -- Ball3/RConn1
  Spatial Contact Force3/LConn1 -- Ball1/RConn1
  Ball8/RConn1 -- Spatial Contact Force4/LConn1
  Ball5/RConn1 -- Spatial Contact Force7/LConn1
  Ball6/RConn1 -- Spatial Contact Force6/LConn1
  Ball7/RConn1 -- Spatial Contact Force5/LConn1
  Ball15/RConn1 -- Spatial Contact Force13/LConn1
  Ball12/RConn1 -- Spatial Contact Force8/LConn1
  Ball9/RConn1 -- Spatial Contact Force11/LConn1
  Ball13/RConn1 -- Spatial Contact Force15/LConn1
  Ball10/RConn1 -- Spatial Contact Force10/LConn1
  Ball14/RConn1 -- Spatial Contact Force14/LConn1
  Ball11/RConn1 -- Spatial Contact Force9/LConn1
  Ball16/RConn1 -- Spatial Contact Force12/LConn1
  Ball18/RConn1 -- Spatial Contact Force16/LConn1
  Ball17/RConn1 -- Spatial Contact Force17/LConn1
  Spatial Contact Force7/RConn1 -- Spatial Contact Force6/RConn1 -- Spatial Contact Force12/RConn1 -- Spatial Contact Force17/RConn1 -- Spatial Contact Force16/RConn1 -- Spatial Contact Force13/RConn1 -- Spatial Contact Force14/RConn1 -- Spatial Contact Force15/RConn1 -- Spatial Contact Force8/RConn1 -- Spatial Contact Force9/RConn1 -- Spatial Contact Force10/RConn1 -- Spatial Contact Force11/RConn1 -- Spatial Contact Force4/RConn1 -- Spatial Contact Force5/RConn1 -- Spatial Contact Force/RConn1 -- Spatial Contact Force1/RConn1 -- Spatial Contact Force2/RConn1 -- G/RConn1 -- Spatial Contact Force3/RConn1

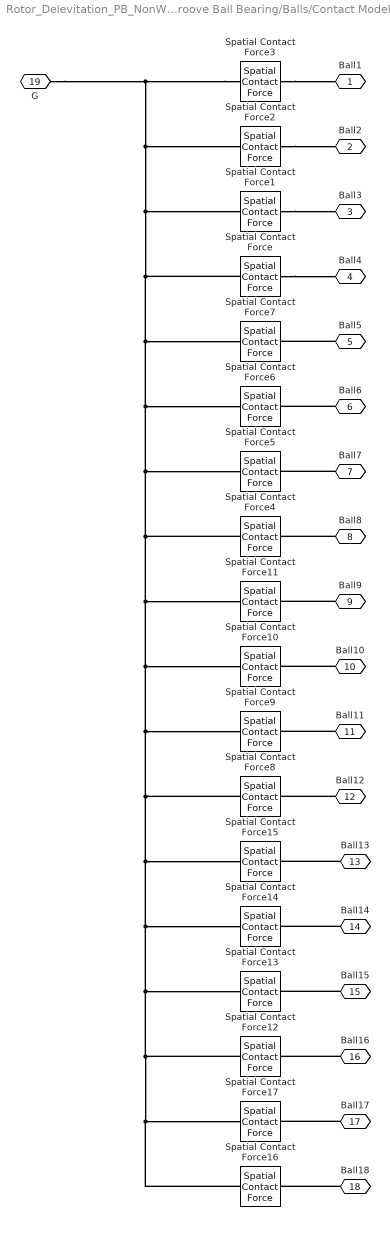
== system Rotor_Delevitation_PB_NonWhirl/Left Deep Groove Ball Bearing/Balls/Contact Modelling1 ==
  Spatial Contact Force{,1..17} (18 alike) : sm_lib/Forces and Torques/Spatial Contact Force  NormalForceType=SmoothSpringDamper  NormalStiffness=1e6  NormalStiffnessUnits=N/m  NormalDamping=1e3  NormalDampingUnits=N/(m/s)  NormalTransitionRegionWidth=1e-4  NormalTransitionRegionWidthUnits=m  FrictionType=SmoothStickSlip  CoefficientOfStaticFriction=0.5  CoefficientOfDynamicFriction=0.3  FrictionalCriticalVelocity=1e-3  FrictionalCriticalVelocityUnits=m/s  SenseContactSignal=off  SensePenetrationDepth=off  SenseSeparationDistance=off  SenseNormalForceMagnitude=off  SenseFrictionalForceMagnitude=off  SenseNormalVelocity=off  SenseTangentialVelocity=off  SenseContactBaseRotation=off  SenseContactBaseTranslation=off  SenseContactFollowerRotation=off  SenseContactFollowerTranslation=off  ZeroCrossDetectContactStartAndEnd=off
  Ball1 : PMIOPort  Side=Right
  Ball2 : PMIOPort  Port=2  Side=Right
  Ball3 : PMIOPort  Port=3  Side=Right
  Ball4 : PMIOPort  Port=4  Side=Right
  Ball5 : PMIOPort  Port=5  Side=Right
  Ball6 : PMIOPort  Port=6  Side=Right
  Ball7 : PMIOPort  Port=7  Side=Right
  Ball8 : PMIOPort  Port=8  Side=Right
  Ball9 : PMIOPort  Port=9  Side=Right
  Ball10 : PMIOPort  Port=10  Side=Right
  Ball11 : PMIOPort  Port=11  Side=Right
  Ball12 : PMIOPort  Port=12  Side=Right
  Ball13 : PMIOPort  Port=13  Side=Right
  Ball14 : PMIOPort  Port=14  Side=Right
  Ball15 : PMIOPort  Port=15  Side=Right
  Ball16 : PMIOPort  Port=16  Side=Right
  Ball17 : PMIOPort  Port=17  Side=Right
  Ball18 : PMIOPort  Port=18  Side=Right
  G : PMIOPort  Port=19  Side=Left
  connections:
  Spatial Contact Force3/RConn1 -- G/RConn1 -- Spatial Contact Force2/RConn1 -- Spatial Contact Force1/RConn1 -- Spatial Contact Force/RConn1 -- Spatial Contact Force5/RConn1 -- Spatial Contact Force4/RConn1 -- Spatial Contact Force11/RConn1 -- Spatial Contact Force10/RConn1 -- Spatial Contact Force9/RConn1 -- Spatial Contact Force8/RConn1 -- Spatial Contact Force15/RConn1 -- Spatial Contact Force14/RConn1 -- Spatial Contact Force13/RConn1 -- Spatial Contact Force16/RConn1 -- Spatial Contact Force17/RConn1 -- Spatial Contact Force12/RConn1 -- Spatial Contact Force6/RConn1 -- Spatial Contact Force7/RConn1
  Ball17/RConn1 -- Spatial Contact Force17/LConn1
  Ball18/RConn1 -- Spatial Contact Force16/LConn1
  Ball16/RConn1 -- Spatial Contact Force12/LConn1
  Ball11/RConn1 -- Spatial Contact Force9/LConn1
  Ball14/RConn1 -- Spatial Contact Force14/LConn1
  Ball10/RConn1 -- Spatial Contact Force10/LConn1
  Ball13/RConn1 -- Spatial Contact Force15/LConn1
  Ball9/RConn1 -- Spatial Contact Force11/LConn1
  Ball12/RConn1 -- Spatial Contact Force8/LConn1
  Ball15/RConn1 -- Spatial Contact Force13/LConn1
  Ball7/RConn1 -- Spatial Contact Force5/LConn1
  Ball6/RConn1 -- Spatial Contact Force6/LConn1
  Ball5/RConn1 -- Spatial Contact Force7/LConn1
  Ball8/RConn1 -- Spatial Contact Force4/LConn1
  Spatial Contact Force3/LConn1 -- Ball1/RConn1
  Spatial Contact Force1/LConn1 -- Ball3/RConn1
  Spatial Contact Force/LConn1 -- Ball4/RConn1
  Spatial Contact Force2/LConn1 -- Ball2/RConn1

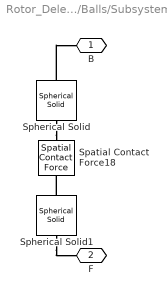
== system Rotor_Delevitation_PB_NonWhirl/Left Deep Groove Ball Bearing/Balls/Subsystem ==
  Spatial Contact Force18 : sm_lib/Forces and Torques/Spatial Contact Force  NormalForceType=SmoothSpringDamper  NormalStiffness=1e6  NormalStiffnessUnits=N/m  NormalDamping=1e3  NormalDampingUnits=N/(m/s)  NormalTransitionRegionWidth=1e-4  NormalTransitionRegionWidthUnits=m  FrictionType=None  CoefficientOfStaticFriction=0.5  CoefficientOfDynamicFriction=0.3  FrictionalCriticalVelocity=1e-3  FrictionalCriticalVelocityUnits=m/s  SenseContactSignal=off  SensePenetrationDepth=off  SenseSeparationDistance=off  SenseNormalForceMagnitude=off  SenseFrictionalForceMagnitude=off  SenseNormalVelocity=off  SenseTangentialVelocity=off  SenseContactBaseRotation=off  SenseContactBaseTranslation=off  SenseContactFollowerRotation=off  SenseContactFollowerTranslation=off  ZeroCrossDetectContactStartAndEnd=off
  Spherical Solid : sm_lib/Body Elements/Spherical Solid  SphereRadius=Cage_R  SphereRadiusUnits=mm  ExportEntireGeometry=on  InertiaType=CalculateFromGeometry  BasedOnType=Density  Density=0  DensityUnits=kg/m^3  Mass=1  MassUnits=kg  CenterOfMass=[0 0 0]  CenterOfMassUnits=m  MomentsOfInertia=[1 1 1]  MomentsOfInertiaUnits=kg*m^2  ProductsOfInertia=[0 0 0]  ProductsOfInertiaUnits=kg*m^2  GraphicType=FromGeometry  MarkerShape=Sphere  MarkerSize=10  GraphicVisPropType=SimpleVisualProperties  GraphicDiffuseColor=[0.5 0.5 0.5]  GraphicOpacity=Cage_opc  GraphicSpecularColor=[0.5 0.5 0.5 1.0]  GraphicAmbientColor=[0.15 0.15 0.15 1.0]  GraphicEmissiveColor=[0.0 0.0 0.0 1.0]  GraphicShininess=75  DoExposeReferenceFrame=on  SerializedFrames=<Frames/>
  Spherical Solid1 : sm_lib/Body Elements/Spherical Solid  SphereRadius=Cage_R  SphereRadiusUnits=mm  ExportEntireGeometry=on  InertiaType=CalculateFromGeometry  BasedOnType=Density  Density=0  DensityUnits=kg/m^3  Mass=1  MassUnits=kg  CenterOfMass=[0 0 0]  CenterOfMassUnits=m  MomentsOfInertia=[1 1 1]  MomentsOfInertiaUnits=kg*m^2  ProductsOfInertia=[0 0 0]  ProductsOfInertiaUnits=kg*m^2  GraphicType=FromGeometry  MarkerShape=Sphere  MarkerSize=10  GraphicVisPropType=SimpleVisualProperties  GraphicDiffuseColor=[0.5 0.5 0.5]  GraphicOpacity=Cage_opc  GraphicSpecularColor=[0.5 0.5 0.5 1.0]  GraphicAmbientColor=[0.15 0.15 0.15 1.0]  GraphicEmissiveColor=[0.0 0.0 0.0 1.0]  GraphicShininess=75  DoExposeReferenceFrame=on  SerializedFrames=<Frames/>
  B : PMIOPort  Side=Left
  F : PMIOPort  Port=2  Side=Right
  connections:
  Spherical Solid1/RConn1 -- F/RConn1
  Spherical Solid1/LConn1 -- Spatial Contact Force18/RConn1
  Spherical Solid/LConn1 -- Spatial Contact Force18/LConn1
  Spherical Solid/RConn1 -- B/RConn1

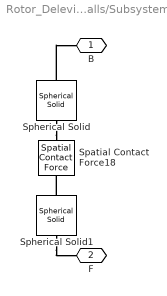
== system Rotor_Delevitation_PB_NonWhirl/Left Deep Groove Ball Bearing/Balls/Subsystem1 ==
  Spatial Contact Force18 : sm_lib/Forces and Torques/Spatial Contact Force  NormalForceType=SmoothSpringDamper  NormalStiffness=1e6  NormalStiffnessUnits=N/m  NormalDamping=1e3  NormalDampingUnits=N/(m/s)  NormalTransitionRegionWidth=1e-4  NormalTransitionRegionWidthUnits=m  FrictionType=None  CoefficientOfStaticFriction=0.5  CoefficientOfDynamicFriction=0.3  FrictionalCriticalVelocity=1e-3  FrictionalCriticalVelocityUnits=m/s  SenseContactSignal=off  SensePenetrationDepth=off  SenseSeparationDistance=off  SenseNormalForceMagnitude=off  SenseFrictionalForceMagnitude=off  SenseNormalVelocity=off  SenseTangentialVelocity=off  SenseContactBaseRotation=off  SenseContactBaseTranslation=off  SenseContactFollowerRotation=off  SenseContactFollowerTranslation=off  ZeroCrossDetectContactStartAndEnd=off
  Spherical Solid : sm_lib/Body Elements/Spherical Solid  SphereRadius=Cage_R  SphereRadiusUnits=mm  ExportEntireGeometry=on  InertiaType=CalculateFromGeometry  BasedOnType=Density  Density=0  DensityUnits=kg/m^3  Mass=1  MassUnits=kg  CenterOfMass=[0 0 0]  CenterOfMassUnits=m  MomentsOfInertia=[1 1 1]  MomentsOfInertiaUnits=kg*m^2  ProductsOfInertia=[0 0 0]  ProductsOfInertiaUnits=kg*m^2  GraphicType=FromGeometry  MarkerShape=Sphere  MarkerSize=10  GraphicVisPropType=SimpleVisualProperties  GraphicDiffuseColor=[0.5 0.5 0.5]  GraphicOpacity=Cage_opc  GraphicSpecularColor=[0.5 0.5 0.5 1.0]  GraphicAmbientColor=[0.15 0.15 0.15 1.0]  GraphicEmissiveColor=[0.0 0.0 0.0 1.0]  GraphicShininess=75  DoExposeReferenceFrame=on  SerializedFrames=<Frames/>
  Spherical Solid1 : sm_lib/Body Elements/Spherical Solid  SphereRadius=Cage_R  SphereRadiusUnits=mm  ExportEntireGeometry=on  InertiaType=CalculateFromGeometry  BasedOnType=Density  Density=0  DensityUnits=kg/m^3  Mass=1  MassUnits=kg  CenterOfMass=[0 0 0]  CenterOfMassUnits=m  MomentsOfInertia=[1 1 1]  MomentsOfInertiaUnits=kg*m^2  ProductsOfInertia=[0 0 0]  ProductsOfInertiaUnits=kg*m^2  GraphicType=FromGeometry  MarkerShape=Sphere  MarkerSize=10  GraphicVisPropType=SimpleVisualProperties  GraphicDiffuseColor=[0.5 0.5 0.5]  GraphicOpacity=Cage_opc  GraphicSpecularColor=[0.5 0.5 0.5 1.0]  GraphicAmbientColor=[0.15 0.15 0.15 1.0]  GraphicEmissiveColor=[0.0 0.0 0.0 1.0]  GraphicShininess=75  DoExposeReferenceFrame=on  SerializedFrames=<Frames/>
  B : PMIOPort  Side=Left
  F : PMIOPort  Port=2  Side=Right
  connections:
  Spherical Solid/RConn1 -- B/RConn1
  Spherical Solid/LConn1 -- Spatial Contact Force18/LConn1
  Spherical Solid1/LConn1 -- Spatial Contact Force18/RConn1
  Spherical Solid1/RConn1 -- F/RConn1

== system Rotor_Delevitation_PB_NonWhirl/Left Deep Groove Ball Bearing/Balls/Subsystem10 ==
  Spatial Contact Force18 : sm_lib/Forces and Torques/Spatial Contact Force  NormalForceType=SmoothSpringDamper  NormalStiffness=1e6  NormalStiffnessUnits=N/m  NormalDamping=1e3  NormalDampingUnits=N/(m/s)  NormalTransitionRegionWidth=1e-4  NormalTransitionRegionWidthUnits=m  FrictionType=None  CoefficientOfStaticFriction=0.5  CoefficientOfDynamicFriction=0.3  FrictionalCriticalVelocity=1e-3  FrictionalCriticalVelocityUnits=m/s  SenseContactSignal=off  SensePenetrationDepth=off  SenseSeparationDistance=off  SenseNormalForceMagnitude=off  SenseFrictionalForceMagnitude=off  SenseNormalVelocity=off  SenseTangentialVelocity=off  SenseContactBaseRotation=off  SenseContactBaseTranslation=off  SenseContactFollowerRotation=off  SenseContactFollowerTranslation=off  ZeroCrossDetectContactStartAndEnd=off
  Spherical Solid : sm_lib/Body Elements/Spherical Solid  SphereRadius=Cage_R  SphereRadiusUnits=mm  ExportEntireGeometry=on  InertiaType=CalculateFromGeometry  BasedOnType=Density  Density=0  DensityUnits=kg/m^3  Mass=1  MassUnits=kg  CenterOfMass=[0 0 0]  CenterOfMassUnits=m  MomentsOfInertia=[1 1 1]  MomentsOfInertiaUnits=kg*m^2  ProductsOfInertia=[0 0 0]  ProductsOfInertiaUnits=kg*m^2  GraphicType=FromGeometry  MarkerShape=Sphere  MarkerSize=10  GraphicVisPropType=SimpleVisualProperties  GraphicDiffuseColor=[0.5 0.5 0.5]  GraphicOpacity=Cage_opc  GraphicSpecularColor=[0.5 0.5 0.5 1.0]  GraphicAmbientColor=[0.15 0.15 0.15 1.0]  GraphicEmissiveColor=[0.0 0.0 0.0 1.0]  GraphicShininess=75  DoExposeReferenceFrame=on  SerializedFrames=<Frames/>
  Spherical Solid1 : sm_lib/Body Elements/Spherical Solid  SphereRadius=Cage_R  SphereRadiusUnits=mm  ExportEntireGeometry=on  InertiaType=CalculateFromGeometry  BasedOnType=Density  Density=0  DensityUnits=kg/m^3  Mass=1  MassUnits=kg  CenterOfMass=[0 0 0]  CenterOfMassUnits=m  MomentsOfInertia=[1 1 1]  MomentsOfInertiaUnits=kg*m^2  ProductsOfInertia=[0 0 0]  ProductsOfInertiaUnits=kg*m^2  GraphicType=FromGeometry  MarkerShape=Sphere  MarkerSize=10  GraphicVisPropType=SimpleVisualProperties  GraphicDiffuseColor=[0.5 0.5 0.5]  GraphicOpacity=Cage_opc  GraphicSpecularColor=[0.5 0.5 0.5 1.0]  GraphicAmbientColor=[0.15 0.15 0.15 1.0]  GraphicEmissiveColor=[0.0 0.0 0.0 1.0]  GraphicShininess=75  DoExposeReferenceFrame=on  SerializedFrames=<Frames/>
  B : PMIOPort  Side=Left
  F : PMIOPort  Port=2  Side=Right
  connections:
  Spherical Solid1/RConn1 -- F/RConn1
  Spherical Solid1/LConn1 -- Spatial Contact Force18/RConn1
  Spherical Solid/LConn1 -- Spatial Contact Force18/LConn1
  Spherical Solid/RConn1 -- B/RConn1
